simulink model "PFC_69C_03_06_V01_3Phase_3_2KW"  (R2022b)
settings: Solver=FixedStepAuto  StartTime=0.0  StopTime=Inf  RelTol=1e-3  EnableMultiTasking=on
model workspace (MAT data in the model file):
  ADC_Gain = 1241.21212121
  DAC_Gain = 0.000805860805861
  Inductor_Current_Divider_Gain_Phase_A = 33.4
  Inductor_Current_Divider_Gain_Phase_B = 33.4
  Vbulk_Divider_Gain = 276.854928018
  Vin_Divider_Gain = 556.17352614
undefined symbols (not defined in the file or in its folder): GPTRIP1SEL, GPTRIP2SEL, SCI_A_Transmit, SCI_A_Transmit_Current_Suffix, SCI_A_Transmit_one_shot_Suffix, SCI_A_Transmit_Polarity_Suffix, SCI_A_Transmit_relay_Suffix, SCI_A_Transmit_Vbulk_Suffix, SCI_A_Transmit_Vin_rms_Suffix, SCI_A_Transmit_Vin_Suffix, SCI_A_Transmit_Vmid_Suffix, SCI_A_Transmit_Vp_Suffix, SCI_A_Transmit_Vpfc_Suffix, TZ1, TZ2
libraries: c280xlib x38, c2802xlib x34, simulink x17, c2000lib x1
(part 4 of 8)

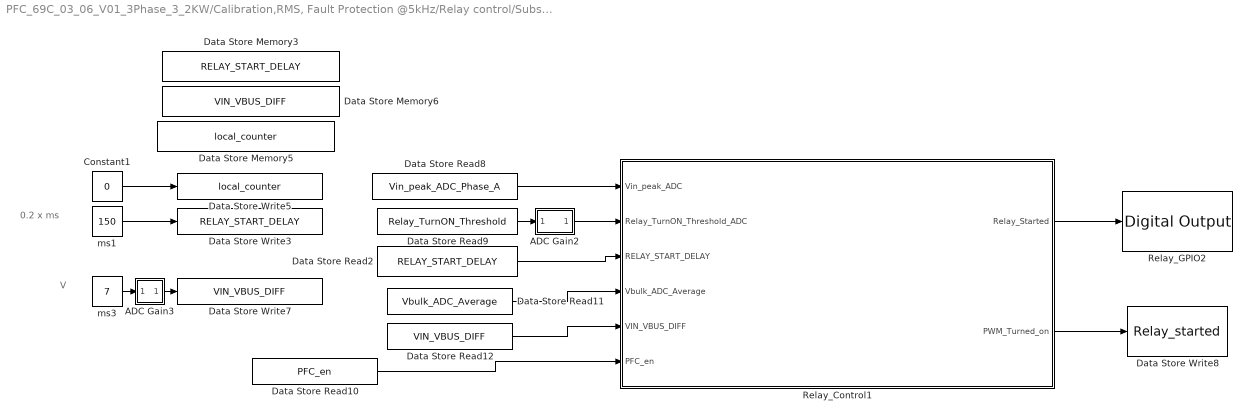
== system PFC_69C_03_06_V01_3Phase_3_2KW/Calibration,RMS, Fault Protection @5kHz/Relay control/Subsystem ==
  note: 0.2 x ms
  note: V
  ADC Gain2 : Subsystem
  ADC Gain3 : Subsystem
  Constant1 : Constant  Value=0
  Data Store Memory3 : DataStoreMemory  DataStoreName=RELAY_START_DELAY  WriteAfterWriteMsg=warning  ShowAdditionalParam=off
  Data Store Memory5 : DataStoreMemory  DataStoreName=local_counter  WriteAfterWriteMsg=warning  ShowAdditionalParam=off
  Data Store Memory6 : DataStoreMemory  DataStoreName=VIN_VBUS_DIFF  WriteAfterWriteMsg=warning  ShowAdditionalParam=off
  Data Store Read10 : DataStoreRead  DataStoreName=PFC_en  IndexOptions=Index vector (dialog)  Indices=1  OutputSizes=1
  Data Store Read11 : DataStoreRead  DataStoreName=Vbulk_ADC_Average  IndexOptions=Index vector (dialog)  Indices=1  OutputSizes=1
  Data Store Read12 : DataStoreRead  DataStoreName=VIN_VBUS_DIFF  IndexOptions=Index vector (dialog)  Indices=1  OutputSizes=1
  Data Store Read2 : DataStoreRead  DataStoreName=RELAY_START_DELAY  IndexOptions=Index vector (dialog)  Indices=1  OutputSizes=1
  Data Store Read8 : DataStoreRead  DataStoreName=Vin_peak_ADC_Phase_A  IndexOptions=Index vector (dialog)  Indices=1  OutputSizes=1
  Data Store Read9 : DataStoreRead  DataStoreName=Relay_TurnON_Threshold  IndexOptions=Index vector (dialog)  Indices=1  OutputSizes=1
  Data Store Write3 : DataStoreWrite  DataStoreName=RELAY_START_DELAY  IndexOptions=Index vector (dialog)  Indices=1  OutputSizes=1
  Data Store Write5 : DataStoreWrite  DataStoreName=local_counter  IndexOptions=Index vector (dialog)  Indices=1  OutputSizes=1
  Data Store Write7 : DataStoreWrite  DataStoreName=VIN_VBUS_DIFF  IndexOptions=Index vector (dialog)  Indices=1  OutputSizes=1
  Data Store Write8 : DataStoreWrite  DataStoreName=Relay_started  IndexOptions=Index vector (dialog)  Indices=1  OutputSizes=1
  Relay_Control1 : Stateflow chart  TreatAsAtomicUnit=on
  Relay_GPIO2 : c280xlib/Digital Output  GPIO_Number=GPIO8~GPIO15  GPIO_Bit0=on  GPIO_BIT0_Toggle=off  GPIO_Bit1=off  GPIO_BIT1_Toggle=off  GPIO_Bit2=off  GPIO_BIT2_Toggle=off  GPIO_Bit3=off  GPIO_BIT3_Toggle=off  GPIO_Bit4=off  GPIO_BIT4_Toggle=off  GPIO_Bit5=off  GPIO_BIT5_Toggle=off  GPIO_Bit6=off  GPIO_BIT6_Toggle=off  GPIO_Bit7=off  GPIO_BIT7_Toggle=off
  ms1 : Constant  Value=150
  ms3 : Constant  Value=7
  wires:
  Data Store Read8/1 -> Relay_Control1/1(Vin_peak_ADC)
  Data Store Read11/1 -> Relay_Control1/4(Vbulk_ADC_Average)
  Relay_Control1/2(PWM_Turned_on) -> Data Store Write8/1
  Data Store Read9/1 -> ADC Gain2/1(In1)
  Data Store Read2/1 -> Relay_Control1/3(RELAY_START_DELAY)
  Data Store Read10/1 -> Relay_Control1/6(PFC_en)
  ADC Gain3/1(Out1) -> Data Store Write7/1
  ms1/1 -> Data Store Write3/1
  ms3/1 -> ADC Gain3/1(In1)
  Relay_Control1/1(Relay_Started) -> Relay_GPIO2/1
  ADC Gain2/1(Out1) -> Relay_Control1/2(Relay_TurnON_Threshold_ADC)
  Constant1/1 -> Data Store Write5/1
  Data Store Read12/1 -> Relay_Control1/5(VIN_VBUS_DIFF)

== system PFC_69C_03_06_V01_3Phase_3_2KW/Calibration,RMS, Fault Protection @5kHz/Relay control_corrected/ADC Gain ==
  In1 : Inport
  Gain : Gain  Commented=on  Gain=ADC_Gain
  Gain1 : Gain  Commented=on  Gain=1/Vin_Divider_Gain
  Gain2 : Gain  Gain=ADC_Gain
  Gain3 : Gain  Gain=1/Vbulk_Divider_Gain
  Out1 : Outport
  wires:
  Gain1/1 -> Gain/1
  Gain3/1 -> Gain2/1
  In1/1 -> Gain3/1
  Gain2/1 -> Out1/1

== system PFC_69C_03_06_V01_3Phase_3_2KW/Calibration,RMS, Fault Protection @5kHz/Relay control_corrected/ADC Gain1 ==
  In1 : Inport
  Gain : Gain  Gain=ADC_Gain
  Gain1 : Gain  Gain=1/Vin_Divider_Gain
  Out1 : Outport
  wires:
  Gain1/1 -> Gain/1
  In1/1 -> Gain1/1
  Gain/1 -> Out1/1

== system PFC_69C_03_06_V01_3Phase_3_2KW/Calibration,RMS, Fault Protection @5kHz/Relay control_corrected/If Action Subsystem3 ==
  Action Port : ActionPort  ActionPortLabel=if(u1==1 & u2==0)
  Constant : Constant
  Digital Output : c280xlib/Digital Output  GPIO_Number=GPIO16~GPIO23  GPIO_Bit0=off  GPIO_BIT0_Toggle=off  GPIO_Bit1=off  GPIO_BIT1_Toggle=off  GPIO_Bit2=off  GPIO_BIT2_Toggle=off  GPIO_Bit3=off  GPIO_BIT3_Toggle=off  GPIO_Bit4=off  GPIO_BIT4_Toggle=off  GPIO_Bit5=off  GPIO_BIT5_Toggle=off  GPIO_Bit6=on  GPIO_BIT6_Toggle=off  GPIO_Bit7=off  GPIO_BIT7_Toggle=off
  wires:
  Constant/1 -> Digital Output/1

== system PFC_69C_03_06_V01_3Phase_3_2KW/Calibration,RMS, Fault Protection @5kHz/Relay control_corrected/If Action Subsystem4 ==
  Action Port : ActionPort  ActionPortLabel=elseif(u1==1 & u2==1)
  Constant : Constant  Value=0
  Digital Output : c280xlib/Digital Output  GPIO_Number=GPIO16~GPIO23  GPIO_Bit0=off  GPIO_BIT0_Toggle=off  GPIO_Bit1=off  GPIO_BIT1_Toggle=off  GPIO_Bit2=off  GPIO_BIT2_Toggle=off  GPIO_Bit3=off  GPIO_BIT3_Toggle=off  GPIO_Bit4=off  GPIO_BIT4_Toggle=off  GPIO_Bit5=off  GPIO_BIT5_Toggle=off  GPIO_Bit6=on  GPIO_BIT6_Toggle=off  GPIO_Bit7=off  GPIO_BIT7_Toggle=off
  wires:
  Constant/1 -> Digital Output/1

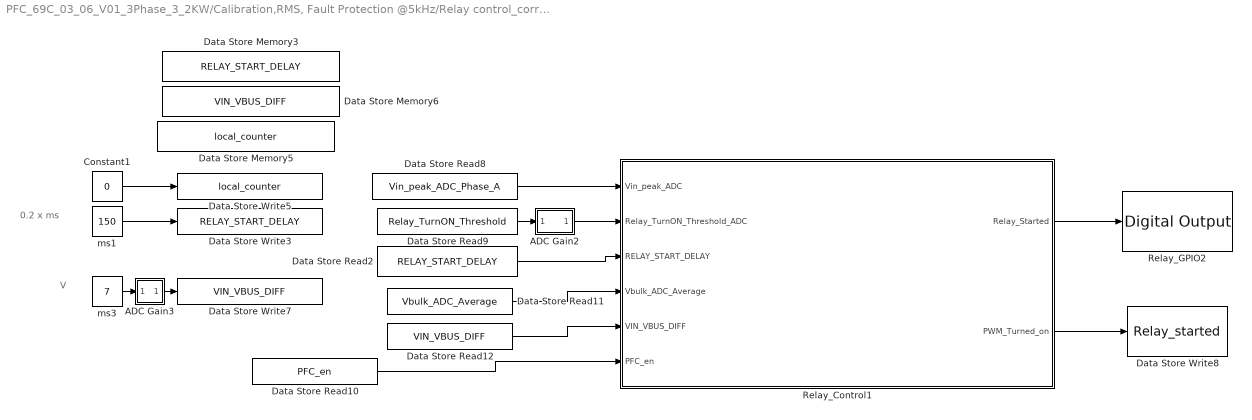
== system PFC_69C_03_06_V01_3Phase_3_2KW/Calibration,RMS, Fault Protection @5kHz/Relay control_corrected/Subsystem ==
  note: 0.2 x ms
  note: V
  ADC Gain2 : Subsystem
  ADC Gain3 : Subsystem
  Constant1 : Constant  Value=0
  Data Store Memory3 : DataStoreMemory  DataStoreName=RELAY_START_DELAY  WriteAfterWriteMsg=warning  ShowAdditionalParam=off
  Data Store Memory5 : DataStoreMemory  DataStoreName=local_counter  WriteAfterWriteMsg=warning  ShowAdditionalParam=off
  Data Store Memory6 : DataStoreMemory  DataStoreName=VIN_VBUS_DIFF  WriteAfterWriteMsg=warning  ShowAdditionalParam=off
  Data Store Read10 : DataStoreRead  DataStoreName=PFC_en  IndexOptions=Index vector (dialog)  Indices=1  OutputSizes=1
  Data Store Read11 : DataStoreRead  DataStoreName=Vbulk_ADC_Average  IndexOptions=Index vector (dialog)  Indices=1  OutputSizes=1
  Data Store Read12 : DataStoreRead  DataStoreName=VIN_VBUS_DIFF  IndexOptions=Index vector (dialog)  Indices=1  OutputSizes=1
  Data Store Read2 : DataStoreRead  DataStoreName=RELAY_START_DELAY  IndexOptions=Index vector (dialog)  Indices=1  OutputSizes=1
  Data Store Read8 : DataStoreRead  DataStoreName=Vin_peak_ADC_Phase_A  IndexOptions=Index vector (dialog)  Indices=1  OutputSizes=1
  Data Store Read9 : DataStoreRead  DataStoreName=Relay_TurnON_Threshold  IndexOptions=Index vector (dialog)  Indices=1  OutputSizes=1
  Data Store Write3 : DataStoreWrite  DataStoreName=RELAY_START_DELAY  IndexOptions=Index vector (dialog)  Indices=1  OutputSizes=1
  Data Store Write5 : DataStoreWrite  DataStoreName=local_counter  IndexOptions=Index vector (dialog)  Indices=1  OutputSizes=1
  Data Store Write7 : DataStoreWrite  DataStoreName=VIN_VBUS_DIFF  IndexOptions=Index vector (dialog)  Indices=1  OutputSizes=1
  Data Store Write8 : DataStoreWrite  DataStoreName=Relay_started  IndexOptions=Index vector (dialog)  Indices=1  OutputSizes=1
  Relay_Control1 : Stateflow chart  TreatAsAtomicUnit=on
  Relay_GPIO2 : c280xlib/Digital Output  GPIO_Number=GPIO8~GPIO15  GPIO_Bit0=on  GPIO_BIT0_Toggle=off  GPIO_Bit1=off  GPIO_BIT1_Toggle=off  GPIO_Bit2=off  GPIO_BIT2_Toggle=off  GPIO_Bit3=off  GPIO_BIT3_Toggle=off  GPIO_Bit4=off  GPIO_BIT4_Toggle=off  GPIO_Bit5=off  GPIO_BIT5_Toggle=off  GPIO_Bit6=off  GPIO_BIT6_Toggle=off  GPIO_Bit7=off  GPIO_BIT7_Toggle=off
  ms1 : Constant  Value=150
  ms3 : Constant  Value=7
  wires:
  Data Store Read8/1 -> Relay_Control1/1(Vin_peak_ADC)
  Data Store Read11/1 -> Relay_Control1/4(Vbulk_ADC_Average)
  Relay_Control1/2(PWM_Turned_on) -> Data Store Write8/1
  Data Store Read9/1 -> ADC Gain2/1(In1)
  Data Store Read2/1 -> Relay_Control1/3(RELAY_START_DELAY)
  Data Store Read10/1 -> Relay_Control1/6(PFC_en)
  ADC Gain3/1(Out1) -> Data Store Write7/1
  ms1/1 -> Data Store Write3/1
  ms3/1 -> ADC Gain3/1(In1)
  Relay_Control1/1(Relay_Started) -> Relay_GPIO2/1
  ADC Gain2/1(Out1) -> Relay_Control1/2(Relay_TurnON_Threshold_ADC)
  Constant1/1 -> Data Store Write5/1
  Data Store Read12/1 -> Relay_Control1/5(VIN_VBUS_DIFF)

== system PFC_69C_03_06_V01_3Phase_3_2KW/Calibration,RMS, Fault Protection @5kHz/Voltage RMS//Averag Calculation/Phase_A ==
  function : TriggerPort  TriggerType=function-call  VariantControl=(inherit)
  Function-Call Generator : simulink/Ports & Subsystems/Function-Call Generator  sample_time=-1  numberOfIterations=1  DisallowWideOutput=off
  Function-Call Split : FunctionCallSplit  IconShape=distinctive  NumOutputPorts=3  OutputPortLayout=default
  RMS Current Calculation_Phase_A : Subsystem  TreatAsAtomicUnit=on
  RMS Voltage Calculation_Phase_A : Subsystem  TreatAsAtomicUnit=on
  Vin_ADC Averaging_Phase_A : Subsystem  TreatAsAtomicUnit=on
  wires:
  Function-Call Generator/1 -> Function-Call Split/1
  Function-Call Split/1 -> RMS Voltage Calculation_Phase_A/Trigger
  Function-Call Split/2 -> RMS Current Calculation_Phase_A/Trigger
  Function-Call Split/3 -> Vin_ADC Averaging_Phase_A/Trigger

== system PFC_69C_03_06_V01_3Phase_3_2KW/Calibration,RMS, Fault Protection @5kHz/Voltage RMS//Averag Calculation/Phase_B ==
  function : TriggerPort  TriggerType=function-call  VariantControl=(inherit)
  Function-Call Generator : simulink/Ports & Subsystems/Function-Call Generator  sample_time=-1  numberOfIterations=1  DisallowWideOutput=off
  Function-Call Split : FunctionCallSplit  IconShape=distinctive  NumOutputPorts=3  OutputPortLayout=default
  RMS Current Calculation_Phase_B : Subsystem  TreatAsAtomicUnit=on
  RMS Voltage Calculation_Phase_B : Subsystem  TreatAsAtomicUnit=on
  Vin_ADC Averaging_Phase_B : Subsystem  TreatAsAtomicUnit=on
  wires:
  Function-Call Split/3 -> Vin_ADC Averaging_Phase_B/Trigger
  Function-Call Split/2 -> RMS Current Calculation_Phase_B/Trigger
  Function-Call Split/1 -> RMS Voltage Calculation_Phase_B/Trigger
  Function-Call Generator/1 -> Function-Call Split/1

== system PFC_69C_03_06_V01_3Phase_3_2KW/Calibration,RMS, Fault Protection @5kHz/Voltage RMS//Averag Calculation/Phase_C ==
  function : TriggerPort  TriggerType=function-call  VariantControl=(inherit)
  Function-Call Generator : simulink/Ports & Subsystems/Function-Call Generator  sample_time=-1  numberOfIterations=1  DisallowWideOutput=off
  Function-Call Split : FunctionCallSplit  IconShape=distinctive  NumOutputPorts=3  OutputPortLayout=default
  RMS Current Calculation_Phase_C : Subsystem  TreatAsAtomicUnit=on
  RMS Voltage Calculation_Phase_C : Subsystem  TreatAsAtomicUnit=on
  Vin_ADC Averaging_Phase_C : Subsystem  TreatAsAtomicUnit=on
  wires:
  Function-Call Generator/1 -> Function-Call Split/1
  Function-Call Split/1 -> RMS Voltage Calculation_Phase_C/Trigger
  Function-Call Split/2 -> RMS Current Calculation_Phase_C/Trigger
  Function-Call Split/3 -> Vin_ADC Averaging_Phase_C/Trigger

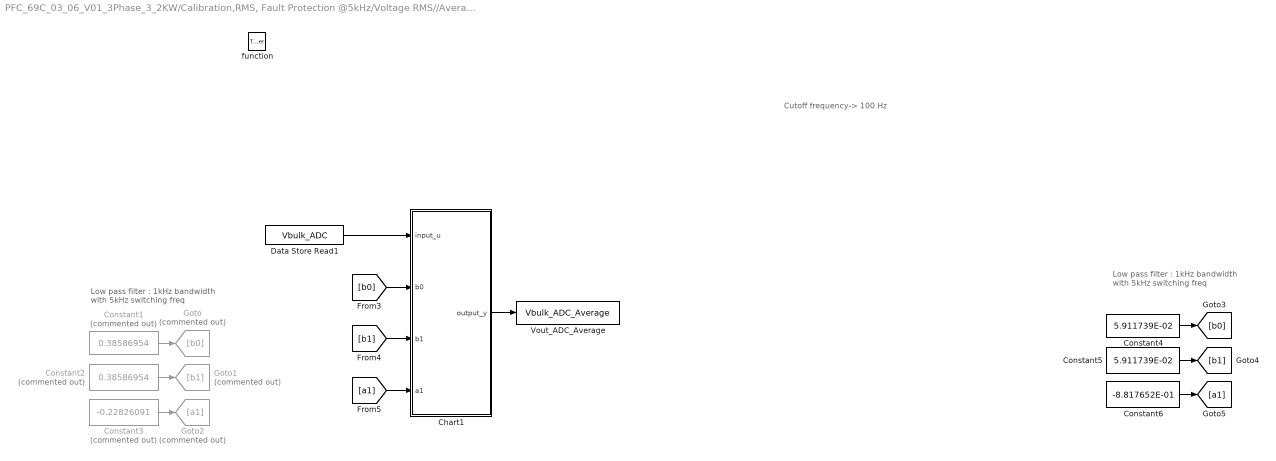
== system PFC_69C_03_06_V01_3Phase_3_2KW/Calibration,RMS, Fault Protection @5kHz/Voltage RMS//Averag Calculation/Vbulk_ADC Averaging ==
  note: Low pass filter :
      | 1kHz bandwidth with 5kHz switching freq
  note: Low pass filter :
      | 1kHz bandwidth with 5kHz switching freq
  note: Cutoff frequency-> 100 Hz
  function : TriggerPort  TriggerType=function-call  VariantControl=(inherit)
  Chart1 : Stateflow chart  TreatAsAtomicUnit=on
  Constant1 : Constant  Commented=on  Value=0.38586954
  Constant2 : Constant  Commented=on  Value=0.38586954
  Constant3 : Constant  Commented=on  Value=-0.22826091
  Constant4 : Constant  Value=5.911739E-02
  Constant5 : Constant  Value=5.911739E-02
  Constant6 : Constant  Value=-8.817652E-01
  Data Store Read1 : DataStoreRead  DataStoreName=Vbulk_ADC  IndexOptions=Index vector (dialog)  Indices=1  OutputSizes=1
  Goto : Goto  Commented=on  GotoTag=b0
  Goto1 : Goto  Commented=on  GotoTag=b1
  Goto2 : Goto  Commented=on  GotoTag=a1
  Vout_ADC_Average : DataStoreWrite  DataStoreName=Vbulk_ADC_Average  IndexOptions=Index vector (dialog)  Indices=1  OutputSizes=1
  wires:
  Chart1/1(output_y) -> Vout_ADC_Average/1
  Data Store Read1/1 -> Chart1/1(input_u)
  [b0] -> Chart1/2(b0)
  [b1] -> Chart1/3(b1)
  [a1] -> Chart1/4(a1)
  Constant2/1 -> Goto1/1
  Constant1/1 -> Goto/1
  Constant3/1 -> Goto2/1
  Constant4/1 -> [b0]
  Constant6/1 -> [a1]
  Constant5/1 -> [b1]

== system PFC_69C_03_06_V01_3Phase_3_2KW/Calibration,RMS, Fault Protection @5kHz/Voltage RMS//Averag Calculation/Vmid_ADC Averaging ==
  note: Low pass filter :
      | 1kHz bandwidth with 5kHz switching freq
  note: Low pass filter :
      | 1kHz bandwidth with 5kHz switching freq
  note: Cutoff frequency-> 100 Hz
  function : TriggerPort  TriggerType=function-call  VariantControl=(inherit)
  Chart1 : Stateflow chart  TreatAsAtomicUnit=on
  Constant1 : Constant  Commented=on  Value=0.38586954
  Constant2 : Constant  Commented=on  Value=0.38586954
  Constant3 : Constant  Commented=on  Value=-0.22826091
  Constant4 : Constant  Value=5.911739E-02
  Constant5 : Constant  Value=5.911739E-02
  Constant6 : Constant  Value=-8.817652E-01
  Data Store Read1 : DataStoreRead  DataStoreName=Vmid_ADC  IndexOptions=Index vector (dialog)  Indices=1  OutputSizes=1
  Goto : Goto  Commented=on  GotoTag=b0
  Goto1 : Goto  Commented=on  GotoTag=b1
  Goto2 : Goto  Commented=on  GotoTag=a1
  Vout_ADC_Average : DataStoreWrite  DataStoreName=Vmid_ADC_Average  IndexOptions=Index vector (dialog)  Indices=1  OutputSizes=1
  wires:
  Chart1/1(output_y) -> Vout_ADC_Average/1
  Data Store Read1/1 -> Chart1/1(input_u)
  [b0] -> Chart1/2(b0)
  [b1] -> Chart1/3(b1)
  [a1] -> Chart1/4(a1)
  Constant2/1 -> Goto1/1
  Constant1/1 -> Goto/1
  Constant3/1 -> Goto2/1
  Constant4/1 -> [b0]
  Constant6/1 -> [a1]
  Constant5/1 -> [b1]

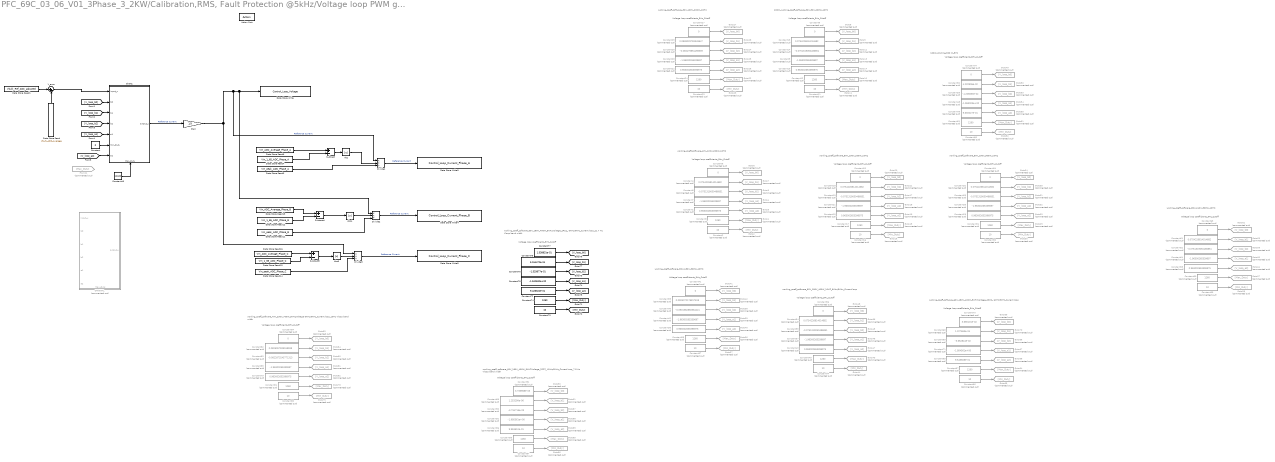
== system PFC_69C_03_06_V01_3Phase_3_2KW/Calibration,RMS, Fault Protection @5kHz/Voltage loop PWM generation (Control)/If Action Subsystem ==
  note: Voltage loop coefficients_5Hz_Cutoff
  note: 100W_Working/200 W_5Hz
  note: 100W_working_coeff_software_30V_90V_200W_10Hz
  note: Voltage loop coefficients_5Hz_Cutoff
  note: Voltage loop coefficients_5Hz_Cutoff
  note: working_coeff_software_30V_100V_200W_10HZ
  note: working_coeff_software_40V_120V_200W_10HZ
  note: Voltage loop coefficients_5Hz_Cutoff
  note: working_coeff_software_50V_150V_200W_10HZ
  note: Voltage loop coefficients_5Hz_Cutoff
  note: working_coeff_software_50V_150V_300W_10HZ
  note: Voltage loop coefficients_5Hz_Cutoff
  note: Voltage loop coefficients_5Hz_Cutoff
  note: working_coeff_software_50V_180V_300W_10HZ
  note: Voltage loop coefficients_5Hz_Cutoff
  note: working_coeff_software_60V_180V_400W_10HZ_6KHz/5KHz_Current loop
  note: Voltage loop coefficients_5Hz_Cutoff
  note: working_coeff_software_80V_240V_500W_10HZ
  note: Voltage loop coefficients_5Hz_Cutoff
  note: working_coeff_software_60V_180V_400W_5KHZVoltage_2P2Z_
      | 6KHz/5KHz_Current loop
  note: working_coeff_software_60V_180V_400W_5KHZVoltage_2P2Z_
      | 6KHz/5KHz_Current loop_21.7 Hz Vloop band width
  note: Voltage loop coefficients_5Hz_Cutoff
  note: Voltage loop coefficients_5Hz_Cutoff
  note: working_coeff_software_70V_230V_700W_5KHZVoltage
      | 6KHz/5KHz_Current loop_10Hz Vloop band width
  note: Voltage loop coefficients_5Hz_Cutoff
  note: working_coeff_software_60V_180V_400W_5KHZVoltage_2P2Z_
      | 6KHz/5KHz_Current loop_7.5 Hz Vloop band width
  Action Port : ActionPort  ActionPortLabel=if((u1==1) & (u2==1))
  Abs : Abs  SaturateOnIntegerOverflow=off
  Abs4 : Abs  SaturateOnIntegerOverflow=off
  Abs5 : Abs  SaturateOnIntegerOverflow=off
  Chart1 : Stateflow chart  TreatAsAtomicUnit=on
      settings: PortSchema="{\"entries\":[{\"content\":{\"sides\":[{\"content\":{\"connectorIds\":[\"In2\",\"In3\",\"In4\",\"In5\",\"In7\",\"In6\",\"In8\"]},\"type\":\"ConnectorPlacement.EquallySpacedRectSide\",\"uuid\":\"98054acb-dc05-45b7-9e49-d1f1309a60af\"},{\"content\":{\"connectorIds\":[\"Out1\"],\"side\":\"RIGHT\"},\"type\":\"ConnectorPlacement.EquallySpacedRectSide\",\"uuid\":\"519c6a11-fba4-4420-9bc2-f24cec898983\"},{\"content\":{\"connectorIds\":[],\"side\":\"TOP\"},\"type\":\"ConnectorPlacement.EquallySpacedRectSide\",\"uuid\":\"37e92206-8070-4c6c-85b3-8eb12c5538cd\"},{\"content\":{\"connectorIds\":[\"In1\"],\"side\":\"BOTTOM\"},\"type\":\"ConnectorPlacement.EquallySpacedRectSide\",\"uuid\":\"a24e42b6-e88f-4c7d-a70a-f75d0d02a985\"}]},\"type\":\"ConnectorPlacement.EquallySpacedConnector\",\"uuid\":\"7d467722-ac20-43d4-98e5-7341f60d2894\"}],\"packageUris\":[\"http://schema.mathworks.com/mf0/Connector/R2020b\"],\"version\":\"1.0\"}"
  Constant : Constant  Value=0
  Constant{1,10,15,22,29,36,43,58,79} (9 alike) : Constant  Commented=on  Value=0.963002653396975
  Constant{2,11,16,23,30,37,44,50,59,66,80,87} (12 alike) : Constant  Commented=on  Value=10  OutDataTypeStr=double
  Constant{3,12,17,24,31,38,45,51,60,67,81,88} (12 alike) : Constant  Commented=on  Value=1260  OutDataTypeStr=double
  Constant{4,13,18,32,54,61} (6 alike) : Constant  Commented=on  Value=0.0754226814014682
  Constant{5,14,19,33,55,62} (6 alike) : Constant  Commented=on  Value=-0.0751319050486851
  Constant{6,8,20,27,34,41,47,56,63,84} (10 alike) : Constant  Commented=on  Value=0
  Constant{7,9,21,28,35,42,57,64,85} (9 alike) : Constant  Commented=on  Value=-1.96300265339697
  Constant25 : Constant  Commented=on  Value=0.0838029793349647
  Constant26 : Constant  Commented=on  Value=-0.083479894498539
  Constant39 : Constant  Commented=on  Value=0.0905072176817619
  Constant40 : Constant  Commented=on  Value=-0.0901582860584221
  Constant46 : Constant  Value=12600
  Constant48 : Constant  Commented=on  Value=-1.963003e+00
  Constant49 : Constant  Commented=on  Value=9.630027e-01
  Constant52 : Constant  Commented=on  Value=4.220906e-02
  Constant53 : Constant  Commented=on  Value=-4.206653e-02
  Constant65 : Constant  Commented=on  Value=9.545608e-01
  Constant68 : Constant  Commented=on  Value=1.227663e-04
  Constant69 : Constant  Commented=on  Value=-3.652824e-02
  Constant70 : Constant  Commented=on  Value=3.665101e-02
  Constant71 : Constant  Commented=on  Value=-1.954561e+00
  Constant72 : Constant  Value=9.426322e-01
  Constant73 : Constant  Value=10  OutDataTypeStr=double
  Constant74 : Constant  Value=1260  OutDataTypeStr=double
  Constant75 : Constant  Value=5.154472e-04
  Constant76 : Constant  Value=-1.533677e-01
  Constant77 : Constant  Value=1.538831e-01
  Constant78 : Constant  Value=-1.942632e+00
  Constant82 : Constant  Commented=on  Value=0.0826057939158938
  Constant83 : Constant  Commented=on  Value=-0.0822873245771313
  Constant86 : Constant  Commented=on  Value=9.953612e-01
  Constant89 : Constant  Commented=on  Value=1.253290e-06
  Constant90 : Constant  Commented=on  Value=-3.734715e-03
  Constant91 : Constant  Commented=on  Value=3.735968e-03
  Constant92 : Constant  Commented=on  Value=-1.995361e+00
  Data Store Read : DataStoreRead  DataStoreName=Vbulk_ADC_Average  IndexOptions=Index vector (dialog)  Indices=1  OutputSizes=1
  Data Store Read1 : DataStoreRead  DataStoreName=Vbulk_Ref_ADC_adjusted  IndexOptions=Index vector (dialog)  Indices=1  OutputSizes=1
  Data Store Read11 : DataStoreRead  DataStoreName=Vin_peak_ADC_Phase_B  IndexOptions=Index vector (dialog)  Indices=1  OutputSizes=1
  Data Store Read12 : DataStoreRead  DataStoreName=Vin_1_65_ADC_Phase_B  IndexOptions=Index vector (dialog)  Indices=1  OutputSizes=1
  Data Store Read13 : DataStoreRead  DataStoreName=Vin_ADC_Average_Phase_B  IndexOptions=Index vector (dialog)  Indices=1  OutputSizes=1
  Data Store Read14 : DataStoreRead  DataStoreName=Vin_peak_ADC_Phase_C  IndexOptions=Index vector (dialog)  Indices=1  OutputSizes=1
  Data Store Read15 : DataStoreRead  DataStoreName=Vin_1_65_ADC_Phase_C  IndexOptions=Index vector (dialog)  Indices=1  OutputSizes=1
  Data Store Read16 : DataStoreRead  DataStoreName=Vin_ADC_Average_Phase_C  IndexOptions=Index vector (dialog)  Indices=1  OutputSizes=1
  Data Store Read3 : DataStoreRead  DataStoreName=Vin_peak_ADC_Phase_A  IndexOptions=Index vector (dialog)  Indices=1  OutputSizes=1
  Data Store Read4 : DataStoreRead  DataStoreName=Vin_1_65_ADC_Phase_A  IndexOptions=Index vector (dialog)  Indices=1  OutputSizes=1
  Data Store Read6 : DataStoreRead  DataStoreName=Vin_ADC_Average_Phase_A  IndexOptions=Index vector (dialog)  Indices=1  OutputSizes=1
  Data Store Write : DataStoreWrite  DataStoreName=Control_Loop_Voltage  IndexOptions=Index vector (dialog)  Indices=1  OutputSizes=1
  Data Store Write3 : DataStoreWrite  DataStoreName=Control_Loop_Current_Phase_A  IndexOptions=Index vector (dialog)  Indices=1  OutputSizes=1
  Data Store Write4 : DataStoreWrite  DataStoreName=Control_Loop_Current_Phase_B  IndexOptions=Index vector (dialog)  Indices=1  OutputSizes=1
  Data Store Write5 : DataStoreWrite  DataStoreName=Control_Loop_Current_Phase_C  IndexOptions=Index vector (dialog)  Indices=1  OutputSizes=1
  Divide1 : Product  Inputs=**/  RndMeth=Zero  SaturateOnIntegerOverflow=on
  Divide2 : Product  Inputs=**/  RndMeth=Zero  SaturateOnIntegerOverflow=on
  Divide3 : Product  Inputs=**/  RndMeth=Zero  SaturateOnIntegerOverflow=on
  From21 : From  Commented=on  GotoTag=Max_Duty
  Gain : Gain  Gain=1/3
  Goto{1,10,15,22,29,36,43,51,57,64,78,85} (12 alike) : Goto  Commented=on  GotoTag=Max_Duty
  Goto{2,11,16,23,30,37,44,52,58,65,79,86} (12 alike) : Goto  Commented=on  GotoTag=Min_Duty
  Goto{3,12,17,24,31,38,45,53,59,66,80,87} (12 alike) : Goto  Commented=on  GotoTag=V_loop_b2
  Goto{4,13,18,25,32,39,46,54,60,67,81,88} (12 alike) : Goto  Commented=on  GotoTag=V_loop_a1
  Goto{5,14,19,26,33,40,47,55,61,68,82,89} (12 alike) : Goto  Commented=on  GotoTag=V_loop_a2
  Goto{6,8,20,27,34,41,48..49,62,69,83,90} (12 alike) : Goto  Commented=on  GotoTag=V_loop_b0
  Goto{7,9,21,28,35,42,50,56,63,70,84,91} (12 alike) : Goto  Commented=on  GotoTag=V_loop_b1
  ORIGINAL : Stateflow chart  Commented=on  TreatAsAtomicUnit=on
      settings: PortSchema="{\"entries\":[{\"content\":{\"sides\":[{\"content\":{\"connectorIds\":[\"In2\",\"In3\",\"In4\",\"In5\",\"In6\",\"In7\"]},\"type\":\"ConnectorPlacement.EquallySpacedRectSide\",\"uuid\":\"98054acb-dc05-45b7-9e49-d1f1309a60af\"},{\"content\":{\"connectorIds\":[\"Out1\"],\"side\":\"RIGHT\"},\"type\":\"ConnectorPlacement.EquallySpacedRectSide\",\"uuid\":\"519c6a11-fba4-4420-9bc2-f24cec898983\"},{\"content\":{\"connectorIds\":[],\"side\":\"TOP\"},\"type\":\"ConnectorPlacement.EquallySpacedRectSide\",\"uuid\":\"37e92206-8070-4c6c-85b3-8eb12c5538cd\"},{\"content\":{\"connectorIds\":[\"In1\"],\"side\":\"BOTTOM\"},\"type\":\"ConnectorPlacement.EquallySpacedRectSide\",\"uuid\":\"a24e42b6-e88f-4c7d-a70a-f75d0d02a985\"}]},\"type\":\"ConnectorPlacement.EquallySpacedConnector\",\"uuid\":\"7d467722-ac20-43d4-98e5-7341f60d2894\"}],\"packageUris\":[\"http://schema.mathworks.com/mf0/Connector/R2020b\"],\"version\":\"1.0\"}"
  Subtract : Sum  Inputs=+-
  Subtract4 : Sum  Inputs=+-
  Subtract5 : Sum  Inputs=+-
  V_error : Sum  Inputs=|+-  AccumDataTypeStr=double  OutDataTypeStr=double
  wires:
  [V_loop_a2] -> Chart1/8(a2)
  Data Store Read/1 -> V_error/2
  Data Store Read1/1 -> V_error/1
  Constant52/1 -> Goto50/1
  Constant51/1 -> Goto51/1
  Constant47/1 -> Goto49/1
  Constant50/1 -> Goto52/1
  Constant49/1 -> Goto55/1
  Constant48/1 -> Goto54/1
  Data Store Read6/1 -> Subtract/1
  Data Store Read4/1 -> Subtract/2
  Subtract/1 -> Abs/1
  Abs/1 -> Divide1/2
  Data Store Read3/1 -> Divide1/3
  Divide1/1 -> Data Store Write3/1  "Reference Current"
  Data Store Read12/1 -> Subtract4/2
  Divide2/1 -> Data Store Write4/1  "Reference Current"
  Data Store Read11/1 -> Divide2/3
  Subtract4/1 -> Abs4/1
  Abs4/1 -> Divide2/2
  Data Store Read13/1 -> Subtract4/1
  Subtract5/1 -> Abs5/1
  Abs5/1 -> Divide3/2
  Data Store Read16/1 -> Subtract5/1
  Data Store Read15/1 -> Subtract5/2
  Data Store Read14/1 -> Divide3/3
  Divide3/1 -> Data Store Write5/1  "Reference Current"
  Constant53/1 -> Goto53/1
  Chart1/1(output_y) -> Gain/1  "Reference Current"
  Constant11/1 -> Goto11/1
  Constant12/1 -> Goto10/1
  Constant10/1 -> Goto14/1
  Constant9/1 -> Goto13/1
  Constant8/1 -> Goto8/1
  Constant13/1 -> Goto9/1
  Constant14/1 -> Goto12/1
  Constant24/1 -> Goto22/1
  Constant28/1 -> Goto25/1
  Constant27/1 -> Goto27/1
  Constant23/1 -> Goto23/1
  Constant22/1 -> Goto26/1
  Constant26/1 -> Goto24/1
  Constant25/1 -> Goto28/1
  Constant1/1 -> Goto5/1
  Constant4/1 -> Goto7/1
  Constant2/1 -> Goto2/1
  Constant6/1 -> Goto6/1
  Constant7/1 -> Goto4/1
  Constant5/1 -> Goto3/1
  Constant3/1 -> Goto1/1
  Constant19/1 -> Goto17/1
  Constant15/1 -> Goto19/1
  Constant21/1 -> Goto18/1
  Constant16/1 -> Goto16/1
  Constant17/1 -> Goto15/1
  Constant20/1 -> Goto20/1
  Constant18/1 -> Goto21/1
  Constant34/1 -> Goto34/1
  Constant35/1 -> Goto32/1
  Constant31/1 -> Goto29/1
  Constant32/1 -> Goto35/1
  Constant29/1 -> Goto33/1
  Constant30/1 -> Goto30/1
  Constant33/1 -> Goto31/1
  Constant39/1 -> Goto42/1
  Constant42/1 -> Goto39/1
  Constant38/1 -> Goto36/1
  Constant37/1 -> Goto37/1
  Constant40/1 -> Goto38/1
  Constant36/1 -> Goto40/1
  Constant41/1 -> Goto41/1
  Constant55/1 -> Goto45/1
  Constant44/1 -> Goto44/1
  Constant45/1 -> Goto43/1
  Constant56/1 -> Goto48/1
  Constant57/1 -> Goto46/1
  Constant54/1 -> Goto56/1
  Constant43/1 -> Goto47/1
  Constant58/1 -> Goto61/1
  Constant63/1 -> Goto62/1
  Constant62/1 -> Goto59/1
  Constant64/1 -> Goto60/1
  Constant61/1 -> Goto63/1
  Constant59/1 -> Goto58/1
  Constant60/1 -> Goto57/1
  Constant65/1 -> Goto68/1
  Constant71/1 -> Goto67/1
  Constant68/1 -> Goto70/1
  Constant70/1 -> Goto69/1
  Constant66/1 -> Goto65/1
  Constant67/1 -> Goto64/1
  Constant69/1 -> Goto66/1
  Constant74/1 -> [Max_Duty]
  Constant76/1 -> [V_loop_b2]
  Constant77/1 -> [V_loop_b0]
  Constant75/1 -> [V_loop_b1]
  Constant73/1 -> [Min_Duty]
  Constant72/1 -> [V_loop_a2]
  Constant78/1 -> [V_loop_a1]
  V_error/1 -> Chart1/2(input_u)
  [V_loop_b0] -> Chart1/3(b0)
  [V_loop_b1] -> Chart1/4(b1)
  [V_loop_b2] -> Chart1/5(b2)
  [V_loop_a1] -> Chart1/7(a1)
  Constant/1 -> Chart1/6(Min_Duty)
  Constant46/1 -> Chart1/1(Max_Duty)
  Constant85/1 -> Goto81/1
  Constant80/1 -> Goto79/1
  Constant84/1 -> Goto83/1
  Constant83/1 -> Goto80/1
  Constant79/1 -> Goto82/1
  Constant81/1 -> Goto78/1
  Constant82/1 -> Goto84/1
  Constant92/1 -> Goto88/1
  Constant89/1 -> Goto91/1
  Constant91/1 -> Goto90/1
  Constant87/1 -> Goto86/1
  Constant90/1 -> Goto87/1
  Constant86/1 -> Goto89/1
  Constant88/1 -> Goto85/1
  Gain/1 -> Divide3/1, Data Store Write/1, Divide2/1, Divide1/1  "Reference Current"

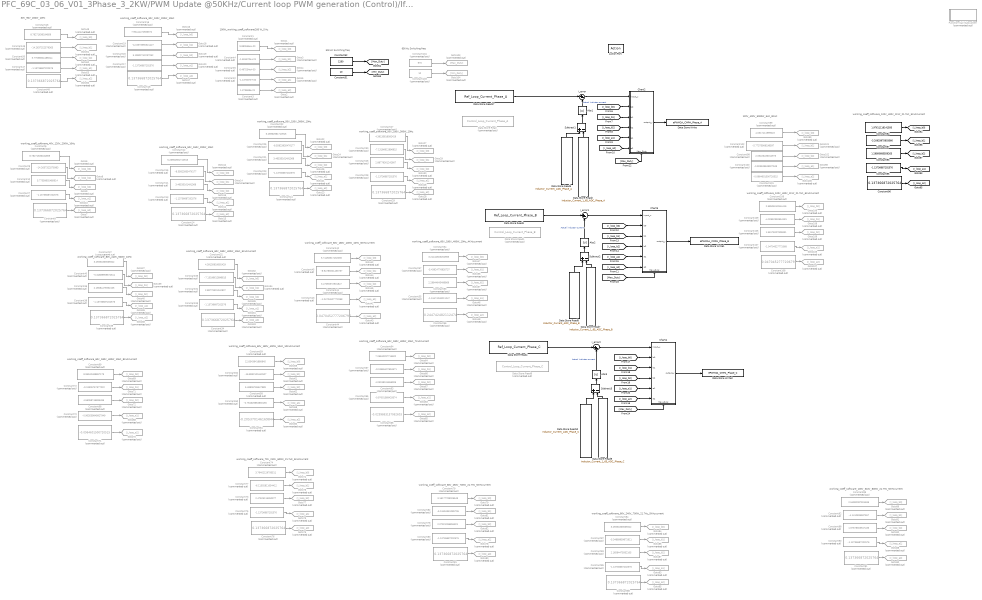
== system PFC_69C_03_06_V01_3Phase_3_2KW/PWM Update @50KHz/Current loop PWM generation (Control)/If Action Subsystem ==
  note: 50KHz Switching freq
  note: 65KHz Switching freq
  note: 30V_90V_200W_10Hz
  note: 100W_working_coeff_software/200 W_5 Hz
  note: working_coeff_software_30V_100V_200W_10Hz
  note: working_coeff_software_40V_120V_200W_10Hz
  note: working_coeff_software_50V_150V_200W_10Hz
  note: working_coeff_software_50V_150V_300W_10Hz
  note: working_coeff_software_50V_180V_300W_10Hz
  note: working_coeff_software_60V_180V_400W_10Hz_5KHzcurrent
  note: working_coeff_software_80V_240V_500W_10Hz
  note: working_coeff_software_60V_180V_400W_10Hz_6KHzcurrent
  note: working_coeff_software_60V_180V_400W_10Hz_4KHzcurrent
  note: working_coeff_software_60V_180V_400W_10Hz_10KHzcurrent
  note: working_coeff_software_60V_180V_400W_10Hz_7KHzcurrent
  note: working_coeff_software_60V_180V_400W_10Hz_8KHzcurrent
  note: working_coeff_software_70V_210V_600W_21.7Hz_5KHzcurrent
  note: working_coeff_software_80V_250V_700W_21.7Hz_5KHzcurrent
  note: working_coeff_software_80V_240V_700W_21.7Hz_5KHzcurrent
  note: working_coeff_software_100V_310V_800W_21.7Hz_5KHzcurrent
  note: working_coeff_software_120V_400V_2KW_21.7Hz_5KHzcurrent
  note: 120V_400V_5000W_5Hz_8KHz
  note: working_coeff_software_120V_400V_2KW_21.7Hz_6KHzcurrent
  Action Port : ActionPort  ActionPortLabel=if((u1 ==1) & (u2==1))
  Abs1 : Abs  SaturateOnIntegerOverflow=off
  Abs2 : Abs  SaturateOnIntegerOverflow=off
  Abs3 : Abs  SaturateOnIntegerOverflow=off
  Chart2 : Stateflow chart  TreatAsAtomicUnit=on
      settings: PortSchema="{\"entries\":[{\"content\":{\"sides\":[{\"content\":{\"connectorIds\":[\"In2\",\"In3\",\"In4\",\"In5\",\"In6\",\"In7\"]},\"type\":\"ConnectorPlacement.EquallySpacedRectSide\",\"uuid\":\"98054acb-dc05-45b7-9e49-d1f1309a60af\"},{\"content\":{\"connectorIds\":[\"Out1\"],\"side\":\"RIGHT\"},\"type\":\"ConnectorPlacement.EquallySpacedRectSide\",\"uuid\":\"519c6a11-fba4-4420-9bc2-f24cec898983\"},{\"content\":{\"connectorIds\":[],\"side\":\"TOP\"},\"type\":\"ConnectorPlacement.EquallySpacedRectSide\",\"uuid\":\"37e92206-8070-4c6c-85b3-8eb12c5538cd\"},{\"content\":{\"connectorIds\":[\"In1\"],\"side\":\"BOTTOM\"},\"type\":\"ConnectorPlacement.EquallySpacedRectSide\",\"uuid\":\"c357f4bc-ad64-4f69-8a5c-2d122a217843\"}]},\"type\":\"ConnectorPlacement.EquallySpacedConnector\",\"uuid\":\"7d467722-ac20-43d4-98e5-7341f60d2894\"}],\"packageUris\":[\"http://schema.mathworks.com/mf0/Connector/R2020b\"],\"version\":\"1.0\"}"
  Chart4 : Stateflow chart  TreatAsAtomicUnit=on
      settings: PortSchema="{\"entries\":[{\"content\":{\"sides\":[{\"content\":{\"connectorIds\":[\"In2\",\"In3\",\"In4\",\"In5\",\"In6\",\"In7\"]},\"type\":\"ConnectorPlacement.EquallySpacedRectSide\",\"uuid\":\"98054acb-dc05-45b7-9e49-d1f1309a60af\"},{\"content\":{\"connectorIds\":[\"Out1\"],\"side\":\"RIGHT\"},\"type\":\"ConnectorPlacement.EquallySpacedRectSide\",\"uuid\":\"519c6a11-fba4-4420-9bc2-f24cec898983\"},{\"content\":{\"connectorIds\":[],\"side\":\"TOP\"},\"type\":\"ConnectorPlacement.EquallySpacedRectSide\",\"uuid\":\"37e92206-8070-4c6c-85b3-8eb12c5538cd\"},{\"content\":{\"connectorIds\":[\"In1\"],\"side\":\"BOTTOM\"},\"type\":\"ConnectorPlacement.EquallySpacedRectSide\",\"uuid\":\"3fbeedd5-4cc1-4149-822b-0a6b54a0fe71\"}]},\"type\":\"ConnectorPlacement.EquallySpacedConnector\",\"uuid\":\"7d467722-ac20-43d4-98e5-7341f60d2894\"}],\"packageUris\":[\"http://schema.mathworks.com/mf0/Connector/R2020b\"],\"version\":\"1.0\"}"
  Chart5 : Stateflow chart  TreatAsAtomicUnit=on
      settings: PortSchema="{\"entries\":[{\"content\":{\"sides\":[{\"content\":{\"connectorIds\":[\"In2\",\"In3\",\"In4\",\"In5\",\"In6\",\"In7\"]},\"type\":\"ConnectorPlacement.EquallySpacedRectSide\",\"uuid\":\"98054acb-dc05-45b7-9e49-d1f1309a60af\"},{\"content\":{\"connectorIds\":[\"Out1\"],\"side\":\"RIGHT\"},\"type\":\"ConnectorPlacement.EquallySpacedRectSide\",\"uuid\":\"519c6a11-fba4-4420-9bc2-f24cec898983\"},{\"content\":{\"connectorIds\":[],\"side\":\"TOP\"},\"type\":\"ConnectorPlacement.EquallySpacedRectSide\",\"uuid\":\"37e92206-8070-4c6c-85b3-8eb12c5538cd\"},{\"content\":{\"connectorIds\":[\"In1\"],\"side\":\"BOTTOM\"},\"type\":\"ConnectorPlacement.EquallySpacedRectSide\",\"uuid\":\"c357f4bc-ad64-4f69-8a5c-2d122a217843\"}]},\"type\":\"ConnectorPlacement.EquallySpacedConnector\",\"uuid\":\"7d467722-ac20-43d4-98e5-7341f60d2894\"}],\"packageUris\":[\"http://schema.mathworks.com/mf0/Connector/R2020b\"],\"version\":\"1.0\"}"
  Constant1 : Constant  Commented=on  Value=9.880556e+00
  Constant10 : Constant  Commented=on  Value=5.77558602485614
  Constant100 : Constant  Commented=on  Value=-0.903539849927949
  Constant101 : Constant  Commented=on  Value=-0.0964601500720515
  Constant102 : Constant  Commented=on  Value=-5.77375908196597
  Constant103 : Constant  Commented=on  Value=10  OutDataTypeStr=double
  Constant104 : Constant  Commented=on  Value=970  OutDataTypeStr=double
  Constant105 : Constant  Commented=on  Value=1.56175007805831
  Constant106 : Constant  Commented=on  Value=2.58506242844416
  Constant107 : Constant  Commented=on  Value=-1.04704527772068
  Constant108 : Constant  Commented=on  Value=0.0470452777206797
  Constant109 : Constant  Commented=on  Value=-4.02652350654181
  Constant11 : Constant  Commented=on  Value=3.46535161491368
  Constant12 : Constant  Commented=on  Value=5.26962981710915
  Constant{7,13,17,23,28,33,38,47,75,80,85,90} (12 alike) : Constant  Commented=on  Value=-1.13736687202576
  Constant{8,14,18,24,29,34,39,48,76,81,86,91} (12 alike) : Constant  Commented=on  Value=0.137366872025764
  Constant15 : Constant  Commented=on  Value=-8.55823935476177
  Constant16 : Constant  Commented=on  Value=7.90444472566372
  Constant19 : Constant  Commented=on  Value=-12.8373590321427
  Constant2 : Constant  Commented=on  Value=-1.137367e+00
  Constant20 : Constant  Commented=on  Value=5.19802742237052
  Constant21 : Constant  Commented=on  Value=3.46535161491368
  Constant22 : Constant  Commented=on  Value=5.26962981710915
  Constant25 : Constant  Commented=on  Value=-8.55823935476177
  Constant26 : Constant  Commented=on  Value=2.88779301242807
  Constant27 : Constant  Commented=on  Value=4.39135818092429
  Constant3 : Constant  Commented=on  Value=1.373669e-01
  Constant30 : Constant  Commented=on  Value=-7.13186612896815
  Constant31 : Constant  Commented=on  Value=2.88779301242807
  Constant32 : Constant  Commented=on  Value=4.39135818092429
  Constant35 : Constant  Commented=on  Value=-7.13186612896815
  Constant36 : Constant  Commented=on  Value=2.16584475932105
  Constant37 : Constant  Commented=on  Value=3.29351863569322
  Constant4 : Constant  Commented=on  Value=-1.604670e+01
  Constant40 : Constant  Commented=on  Value=-5.34889959672611
  Constant41 : Constant  Commented=on  Value=3.47055572901847
  Constant42 : Constant  Commented=on  Value=5.74458317432036
  Constant43 : Constant  Commented=on  Value=-1.04704527772068
  Constant44 : Constant  Commented=on  Value=0.0470452777206797
  Constant45 : Constant  Commented=on  Value=-8.94783001453737
  Constant46 : Constant  Commented=on  Value=8.78271636184859
  Constant49 : Constant  Commented=on  Value=-14.2637322579363
  Constant5 : Constant  Commented=on  Value=6.497534e+00
  Constant50 : Constant  Commented=on  Value=5.77558602485614
  Constant51 : Constant  Value=10  OutDataTypeStr=double
  Constant52 : Constant  Value=1260  OutDataTypeStr=double
  Constant53 : Constant  Commented=on  Value=2.29844645486869
  Constant54 : Constant  Commented=on  Value=3.21242603252965
  Constant55 : Constant  Commented=on  Value=-1.24474248211247
  Constant56 : Constant  Commented=on  Value=0.244742482112474
  Constant57 : Constant  Commented=on  Value=-5.43924776835737
  Constant58 : Constant  Commented=on  Value=5.48806736547989
  Constant59 : Constant  Commented=on  Value=12.8343941880845
  Constant6 : Constant  Commented=on  Value=8.78271636184859
  Constant60 : Constant  Commented=on  Value=-0.794629853830155
  Constant61 : Constant  Commented=on  Value=-0.205370146169844
  Constant62 : Constant  Commented=on  Value=-16.8832100442507
  Constant63 : Constant  Commented=on  Value=4.03198104656906
  Constant64 : Constant  Commented=on  Value=7.26840297715602
  Constant65 : Constant  Commented=on  Value=-0.97001368429374
  Constant66 : Constant  Commented=on  Value=-0.0299863157062603
  Constant67 : Constant  Commented=on  Value=-10.8565407694571
  Constant68 : Constant  Commented=on  Value=4.56058746695496
  Constant69 : Constant  Commented=on  Value=8.95942488867179
  Constant70 : Constant  Commented=on  Value=-0.903539849927949
  Constant71 : Constant  Commented=on  Value=-0.0964601500720515
  Constant72 : Constant  Commented=on  Value=-12.8305757377022
  Constant73 : Constant  Commented=on  Value=2.47525115350977
  Constant74 : Constant  Commented=on  Value=3.76402129793511
  Constant77 : Constant  Commented=on  Value=-6.11302811054412
  Constant78 : Constant  Commented=on  Value=2.07921096894821
  Constant79 : Constant  Commented=on  Value=3.16177789026549
  Constant82 : Constant  Commented=on  Value=-5.13494361285706
  Constant83 : Constant  Commented=on  Value=2.16584475932105
  Constant84 : Constant  Commented=on  Value=3.29351863569322
  Constant87 : Constant  Commented=on  Value=-5.34889959672611
  Constant88 : Constant  Commented=on  Value=1.67678303947436
  Constant89 : Constant  Commented=on  Value=2.54982087924636
  Constant9 : Constant  Commented=on  Value=-14.2637322579363
  Constant92 : Constant  Commented=on  Value=-4.1410835587557
  Constant93 : Constant  Value=1.29950685559263
  Constant94 : Constant  Value=1.97611118141593
  Constant95 : Constant  Value=-1.13736687202576
  Constant96 : Constant  Value=0.137366872025764
  Constant97 : Constant  Value=-3.20933975803566
  Constant98 : Constant  Commented=on  Value=2.05226436012973
  Constant99 : Constant  Commented=on  Value=4.0317411999023
  Data Store Read : DataStoreRead  Commented=on  DataStoreName=Control_Loop_Current_Phase_A  IndexOptions=Index vector (dialog)  Indices=1  OutputSizes=1
  Data Store Read1 : DataStoreRead  Commented=on  DataStoreName=Control_Loop_Current_Phase_B  IndexOptions=Index vector (dialog)  Indices=1  OutputSizes=1
  Data Store Read10 : DataStoreRead  DataStoreName=Inductor_Current_ADC_Phase_C  IndexOptions=Index vector (dialog)  Indices=1  OutputSizes=1
  Data Store Read17 : DataStoreRead  DataStoreName=Ref_Loop_Current_Phase_A  IndexOptions=Index vector (dialog)  Indices=1  OutputSizes=1
  Data Store Read2 : DataStoreRead  DataStoreName=Inductor_Current_1_65_ADC_Phase_A  IndexOptions=Index vector (dialog)  Indices=1  OutputSizes=1
  Data Store Read3 : DataStoreRead  DataStoreName=Ref_Loop_Current_Phase_B  IndexOptions=Index vector (dialog)  Indices=1  OutputSizes=1
  Data Store Read4 : DataStoreRead  DataStoreName=Ref_Loop_Current_Phase_C  IndexOptions=Index vector (dialog)  Indices=1  OutputSizes=1
  Data Store Read5 : DataStoreRead  DataStoreName=Inductor_Current_ADC_Phase_A  IndexOptions=Index vector (dialog)  Indices=1  OutputSizes=1
  Data Store Read6 : DataStoreRead  Commented=on  DataStoreName=Control_Loop_Current_Phase_C  IndexOptions=Index vector (dialog)  Indices=1  OutputSizes=1
  Data Store Read7 : DataStoreRead  DataStoreName=Inductor_Current_1_65_ADC_Phase_B  IndexOptions=Index vector (dialog)  Indices=1  OutputSizes=1
  Data Store Read8 : DataStoreRead  DataStoreName=Inductor_Current_ADC_Phase_B  IndexOptions=Index vector (dialog)  Indices=1  OutputSizes=1
  Data Store Read9 : DataStoreRead  DataStoreName=Inductor_Current_1_65_ADC_Phase_C  IndexOptions=Index vector (dialog)  Indices=1  OutputSizes=1
  Data Store Write : DataStoreWrite  DataStoreName=ePWM2A_CMPA_Phase_A  IndexOptions=Index vector (dialog)  Indices=1  OutputSizes=1
  Data Store Write1 : DataStoreWrite  DataStoreName=ePWM1A_CMPA_Phase_B  IndexOptions=Index vector (dialog)  Indices=1  OutputSizes=1
  Data Store Write2 : DataStoreWrite  DataStoreName=ePWM3A_CMPA_Phase_C  IndexOptions=Index vector (dialog)  Indices=1  OutputSizes=1
  Function-Call Subsystem : Subsystem  Commented=on  TreatAsAtomicUnit=on
  Goto{1,6,12,16,22,27,32,37,42,47,49,59,64,69,74,79,84,89,99,106} (20 alike) : Goto  Commented=on  GotoTag=I_loop_b0
  Goto{5,10..11,20..21,26,31,36,41,46,53,58,63,68,73,78,83,88,98,105} (20 alike) : Goto  Commented=on  GotoTag=I_loop_a1
  Goto{2,7,13,17,23,28,33,38,43,48,50,60,65,70,75,80,85,90,100,107} (20 alike) : Goto  Commented=on  GotoTag=I_loop_a2
  Goto{3,8,14,18,24,29,34,39,44,51,56,61,66,71,76,81,86,91,101,108} (20 alike) : Goto  Commented=on  GotoTag=I_loop_b1
  Goto{4,9,15,19,25,30,35,40,45,52,57,62,67,72,77,82,87,92,102,109} (20 alike) : Goto  Commented=on  GotoTag=I_loop_b2
  Goto103 : Goto  Commented=on  GotoTag=Max_Duty
  Goto104 : Goto  Commented=on  GotoTag=Min_Duty
  I_error : Sum  Inputs=|+-  AccumDataTypeStr=double  OutDataTypeStr=double
  I_error1 : Sum  Inputs=|+-  AccumDataTypeStr=double  OutDataTypeStr=double
  I_error2 : Sum  Inputs=|+-  AccumDataTypeStr=double  OutDataTypeStr=double
  Subtract1 : Sum  Inputs=+-
  Subtract2 : Sum  Inputs=+-
  Subtract3 : Sum  Inputs=+-
  wires:
  [I_loop_b2] -> Chart2/5(b2)
  [I_loop_a2] -> Chart2/7(a2)
  [I_loop_b0] -> Chart2/3(b0)
  Subtract1/1 -> Abs1/1
  Data Store Read5/1 -> Subtract1/1
  [I_loop_b1] -> Chart2/4(b1)
  Abs1/1 -> I_error/2  "Actual inductor current"
  I_error/1 -> Chart2/2(input_u)
  [I_loop_a1] -> Chart2/6(a1)
  Data Store Read2/1 -> Subtract1/2
  Chart2/1(output_y) -> Data Store Write/1
  I_error1/1 -> Chart5/2(input_u)
  [I_loop_a1] -> Chart5/6(a1)
  [I_loop_b1] -> Chart5/4(b1)
  Abs2/1 -> I_error1/2  "Actual inductor current"
  Subtract2/1 -> Abs2/1
  [I_loop_b0] -> Chart5/3(b0)
  [I_loop_a2] -> Chart5/7(a2)
  [I_loop_b2] -> Chart5/5(b2)
  Data Store Read8/1 -> Subtract2/1
  Data Store Read7/1 -> Subtract2/2
  Chart4/1(output_y) -> Data Store Write2/1
  I_error2/1 -> Chart4/2(input_u)
  [I_loop_a1] -> Chart4/6(a1)
  [I_loop_b1] -> Chart4/4(b1)
  Abs3/1 -> I_error2/2  "Actual inductor current"
  Subtract3/1 -> Abs3/1
  [I_loop_b0] -> Chart4/3(b0)
  [I_loop_a2] -> Chart4/7(a2)
  [I_loop_b2] -> Chart4/5(b2)
  Data Store Read10/1 -> Subtract3/1
  Data Store Read9/1 -> Subtract3/2
  [Max_Duty] -> Chart2/1(Max_Duty)
  [Max_Duty] -> Chart4/1(Max_Duty)
  Chart5/1(output_y) -> Data Store Write1/1
  [Max_Duty] -> Chart5/1(Max_Duty)
  Constant47/1 -> Goto53/1
  Constant46/1 -> Goto49/1
  Constant49/1 -> Goto51/1
  Constant48/1 -> Goto50/1
  Constant50/1 -> Goto52/1
  Constant51/1 -> [Min_Duty]
  Constant52/1 -> [Max_Duty]
  Data Store Read17/1 -> I_error/1
  Data Store Read3/1 -> I_error1/1
  Data Store Read4/1 -> I_error2/1
  Constant4/1 -> Goto3/1
  Constant1/1 -> Goto1/1
  Constant3/1 -> Goto2/1
  Constant5/1 -> Goto4/1
  Constant2/1 -> Goto5/1
  Constant17/1 -> Goto20/1
  Constant19/1 -> Goto18/1
  Constant16/1 -> Goto16/1
  Constant18/1 -> Goto17/1
  Constant20/1 -> Goto19/1
  Constant7/1 -> Goto10/1
  Constant9/1 -> Goto8/1
  Constant6/1 -> Goto6/1
  Constant8/1 -> Goto7/1
  Constant10/1 -> Goto9/1
  Constant13/1 -> Goto11/1
  Constant11/1 -> Goto15/1
  Constant15/1 -> Goto14/1
  Constant14/1 -> Goto13/1
  Constant12/1 -> Goto12/1
  Constant21/1 -> Goto25/1
  Constant24/1 -> Goto23/1
  Constant23/1 -> Goto21/1
  Constant25/1 -> Goto24/1
  Constant22/1 -> Goto22/1
  Constant30/1 -> Goto29/1
  Constant27/1 -> Goto27/1
  Constant29/1 -> Goto28/1
  Constant28/1 -> Goto26/1
  Constant26/1 -> Goto30/1
  Constant31/1 -> Goto35/1
  Constant33/1 -> Goto31/1
  Constant35/1 -> Goto34/1
  Constant32/1 -> Goto32/1
  Constant34/1 -> Goto33/1
  Constant40/1 -> Goto39/1
  Constant39/1 -> Goto38/1
  Constant36/1 -> Goto40/1
  Constant37/1 -> Goto37/1
  Constant38/1 -> Goto36/1
  Constant42/1 -> Goto42/1
  Constant43/1 -> Goto41/1
  Constant45/1 -> Goto44/1
  Constant41/1 -> Goto45/1
  Constant44/1 -> Goto43/1
  Constant55/1 -> Goto46/1
  Constant54/1 -> Goto47/1
  Constant57/1 -> Goto56/1
  Constant53/1 -> Goto57/1
  Constant56/1 -> Goto48/1
  Constant59/1 -> Goto59/1
  Constant62/1 -> Goto61/1
  Constant58/1 -> Goto62/1
  Constant60/1 -> Goto58/1
  Constant61/1 -> Goto60/1
  Constant66/1 -> Goto65/1
  Constant63/1 -> Goto67/1
  Constant65/1 -> Goto63/1
  Constant67/1 -> Goto66/1
  Constant64/1 -> Goto64/1
  Constant69/1 -> Goto69/1
  Constant70/1 -> Goto68/1
  Constant71/1 -> Goto70/1
  Constant68/1 -> Goto72/1
  Constant72/1 -> Goto71/1
  Constant75/1 -> Goto73/1
  Constant76/1 -> Goto75/1
  Constant77/1 -> Goto76/1
  Constant73/1 -> Goto77/1
  Constant74/1 -> Goto74/1
  Constant78/1 -> Goto82/1
  Constant80/1 -> Goto78/1
  Constant82/1 -> Goto81/1
  Constant81/1 -> Goto80/1
  Constant79/1 -> Goto79/1
  Constant83/1 -> Goto87/1
  Constant85/1 -> Goto83/1
  Constant86/1 -> Goto85/1
  Constant87/1 -> Goto86/1
  Constant84/1 -> Goto84/1
  Constant88/1 -> Goto92/1
  Constant90/1 -> Goto88/1
  Constant91/1 -> Goto90/1
  Constant92/1 -> Goto91/1
  Constant89/1 -> Goto89/1
  Constant93/1 -> [I_loop_b2]
  Constant94/1 -> [I_loop_b0]
  Constant97/1 -> [I_loop_b1]
  Constant96/1 -> [I_loop_a2]
  Constant95/1 -> [I_loop_a1]
  Constant98/1 -> Goto102/1
  Constant100/1 -> Goto98/1
  Constant102/1 -> Goto101/1
  Constant101/1 -> Goto100/1
  Constant99/1 -> Goto99/1
  Constant103/1 -> Goto104/1
  Constant104/1 -> Goto103/1
  Constant108/1 -> Goto107/1
  Constant109/1 -> Goto108/1
  Constant105/1 -> Goto109/1
  Constant107/1 -> Goto105/1
  Constant106/1 -> Goto106/1

== system PFC_69C_03_06_V01_3Phase_3_2KW/PWM Update @50KHz/Fixed Duty update_Phase_A/Archive ==
  Constant : Constant  Value=100
  Data Store Read : DataStoreRead  DataStoreName=Polarity_Phase_A  IndexOptions=Index vector (dialog)  Indices=1  OutputSizes=1
  Data Store Read1 : DataStoreRead  DataStoreName=Near_Zero_Bar_Phase_A  IndexOptions=Index vector (dialog)  Indices=1  OutputSizes=1
  Data Store Read2 : DataStoreRead  DataStoreName=PWM_Duty_UART  IndexOptions=Index vector (dialog)  Indices=1  OutputSizes=1
  Data Store Read5 : DataStoreRead  DataStoreName=Near_Zero_Bar_Phase_A  IndexOptions=Index vector (dialog)  Indices=1  OutputSizes=1
  Data Store Write : DataStoreWrite  DataStoreName=PWM_Duty  IndexOptions=Index vector (dialog)  Indices=1  OutputSizes=1
  If : If  IfExpression=u1 ==1
  If Action Subsystem : Subsystem  TreatAsAtomicUnit=on
  If Action Subsystem1 : Subsystem  TreatAsAtomicUnit=on
  If Action Subsystem2 : Subsystem  TreatAsAtomicUnit=on
  If Action Subsystem3 : Subsystem  TreatAsAtomicUnit=on
  If1 : If  IfExpression=u1 ==0
  Merge : Merge
  Product : Product
  Subtract : Sum  Inputs=-+
  wires:
  If/1 -> If Action Subsystem1/Action
  Data Store Read2/1 -> If Action Subsystem1/1(In1), Subtract/1, Data Store Write/1
  Merge/1 -> Product/2
  If Action Subsystem2/1(Out1) -> Merge/2
  Constant/1 -> Subtract/2
  Data Store Read/1 -> If/1
  Subtract/1 -> If Action Subsystem2/1(In1)
  Data Store Read1/1 -> Product/1
  If/2 -> If Action Subsystem2/Action
  If Action Subsystem1/1(Out1) -> Merge/1
  If1/1 -> If Action Subsystem/Action
  Data Store Read5/1 -> If1/1
  If1/2 -> If Action Subsystem3/Action

== system PFC_69C_03_06_V01_3Phase_3_2KW/PWM Update @50KHz/Fixed Duty update_Phase_A/Subsystem1 ==
  Frequency(kHz) : Inport
  Duty(%) : Inport  Port=2
  Constant1 : Constant  Value=90E6
  Divide : Product  Inputs=*/  RndMeth=Zero  SaturateOnIntegerOverflow=on
  Gain : Gain  Gain=1000
  Gain1 : Gain  Gain=1/100
  Gain2 : Gain  Gain=0.5
  Product1 : Product
  Out1 : Outport
  Out2 : Outport  Port=2
  Out3 : Outport  Port=3
  wires:
  Gain2/1 -> Out3/1
  Gain1/1 -> Product1/2
  Product1/1 -> Gain2/1, Out2/1
  Duty(%)/1 -> Gain1/1
  Divide/1 -> Out1/1, Product1/1
  Gain/1 -> Divide/2
  Constant1/1 -> Divide/1
  Frequency(kHz)/1 -> Gain/1

== system PFC_69C_03_06_V01_3Phase_3_2KW/PWM Update @50KHz/Fixed Duty update_Phase_B_Test/Archive ==
  Constant : Constant  Value=100
  Data Store Read : DataStoreRead  DataStoreName=Polarity_Phase_A  IndexOptions=Index vector (dialog)  Indices=1  OutputSizes=1
  Data Store Read1 : DataStoreRead  DataStoreName=Near_Zero_Bar_Phase_A  IndexOptions=Index vector (dialog)  Indices=1  OutputSizes=1
  Data Store Read2 : DataStoreRead  DataStoreName=PWM_Duty_UART  IndexOptions=Index vector (dialog)  Indices=1  OutputSizes=1
  Data Store Read5 : DataStoreRead  DataStoreName=Near_Zero_Bar_Phase_A  IndexOptions=Index vector (dialog)  Indices=1  OutputSizes=1
  Data Store Write : DataStoreWrite  DataStoreName=PWM_Duty  IndexOptions=Index vector (dialog)  Indices=1  OutputSizes=1
  If : If  IfExpression=u1 ==1
  If Action Subsystem : Subsystem  TreatAsAtomicUnit=on
  If Action Subsystem1 : Subsystem  TreatAsAtomicUnit=on
  If Action Subsystem2 : Subsystem  TreatAsAtomicUnit=on
  If Action Subsystem3 : Subsystem  TreatAsAtomicUnit=on
  If1 : If  IfExpression=u1 ==0
  Merge : Merge
  Product : Product
  Subtract : Sum  Inputs=-+
  wires:
  If/1 -> If Action Subsystem1/Action
  Data Store Read2/1 -> If Action Subsystem1/1(In1), Subtract/1, Data Store Write/1
  Merge/1 -> Product/2
  If Action Subsystem2/1(Out1) -> Merge/2
  Constant/1 -> Subtract/2
  Data Store Read/1 -> If/1
  Subtract/1 -> If Action Subsystem2/1(In1)
  Data Store Read1/1 -> Product/1
  If/2 -> If Action Subsystem2/Action
  If Action Subsystem1/1(Out1) -> Merge/1
  If1/1 -> If Action Subsystem/Action
  Data Store Read5/1 -> If1/1
  If1/2 -> If Action Subsystem3/Action

== system PFC_69C_03_06_V01_3Phase_3_2KW/PWM Update @50KHz/Fixed Duty update_Phase_B_Test/Subsystem1 ==
  Frequency(kHz) : Inport
  Duty(%) : Inport  Port=2
  Constant1 : Constant  Value=90E6
  Divide : Product  Inputs=*/  RndMeth=Zero  SaturateOnIntegerOverflow=on
  Gain : Gain  Gain=1000
  Gain1 : Gain  Gain=1/100
  Gain2 : Gain  Gain=0.5
  Product1 : Product
  Out1 : Outport
  Out2 : Outport  Port=2
  Out3 : Outport  Port=3
  wires:
  Gain2/1 -> Out3/1
  Gain1/1 -> Product1/2
  Product1/1 -> Gain2/1, Out2/1
  Duty(%)/1 -> Gain1/1
  Divide/1 -> Out1/1, Product1/1
  Gain/1 -> Divide/2
  Constant1/1 -> Divide/1
  Frequency(kHz)/1 -> Gain/1
